simulink model "p2Sim"  (R2020a)
settings: Solver=ode3  StartTime=0.0  StopTime=simPrm.tEnd  FixedStep=simPrm.dt  RelTol=1e-3
values from neighbouring files (symbols this model uses):
  denG = [1 4 25]    [p2Setup.m]
  denH = [Tau, 1]    [p2Setup.m]
  numG = 25    [p2Setup.m]
  numH = 1    [p2Setup.m]
  Umax = 2.5    [p2Setup.m]
  Umin = -2.5    [p2Setup.m]
undefined symbols (not defined in the file or in its folder): cl, Control, dend, Discrete, Input, numd, Time
libraries: simulink x1, ctrlSharedLib x1
settings Model: Creator=vmali  LastModifiedBy=vmali
settings DataIOCC: SignalLoggingName=sdata

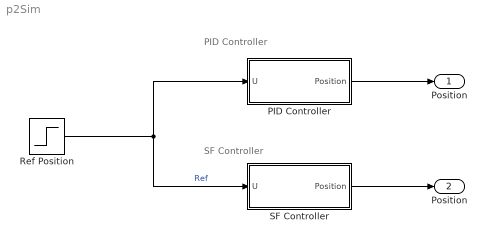
== system p2Sim ==
  note: SF Controller
  note: PID Controller
  PID Controller : Subsystem
  Ref Position : Step  Time=Input.Ts  After=Input.U  SampleTime=0
  SF Controller : Subsystem
  Position : Outport
  "Position " : Outport  Port=2
  wires:
  PID Controller/1(Position) -> Position/1
  SF Controller/1(Position) -> "Position "/1
  Ref Position/1 -> SF Controller/1(U), PID Controller/1(U)  "Ref"

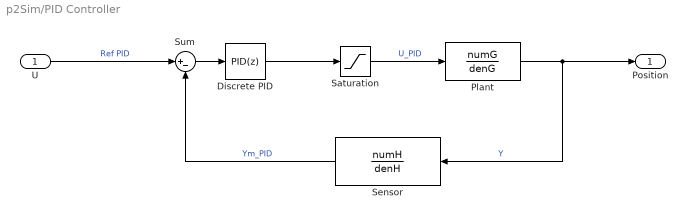
== system p2Sim/PID Controller ==
  U : Inport
  Discrete PID : simulink/Continuous/PID Controller  Controller=PID  Form=Parallel  TimeDomain=Discrete-time  UseExternalTs=off  SampleTime=Control.Z  IntegratorMethod=Forward Euler  FilterMethod=Forward Euler  ControllerParametersSource=internal  P=Control.Kp  I=Control.Ki  D=Control.Kd  UseFilter=on  N=100  TunerSelectOption=Transfer Function Based (PID Tuner App)  InitialConditionSource=internal  InitialConditionForIntegrator=0  InitialConditionForFilter=0  DifferentiatorICPrevScaledInput=0  ExternalReset=none  TrackingMode=off  Kt=1  LimitOutput=off  UpperSaturationLimit=inf  LowerSaturationLimit=-inf  LinearizeAsGain=on  AntiWindupMode=none  Kb=1  POutMin=[]  POutMax=[]  IOutMin=[]  IOutMax=[]  DOutMin=[]  DOutMax=[]  NOutMin=[]  NOutMax=[]  SumOutMin=[]  SumOutMax=[]  SaturationOutMin=[]  SaturationOutMax=[]  PParamMin=[]  PParamMax=[]  IParamMin=[]  IParamMax=[]  DParamMin=[]  DParamMax=[]  NParamMin=[]  NParamMax=[]  KbParamMin=[]  KbParamMax=[]  KtParamMin=[]  KtParamMax=[]  KbOutMin=[]  KbOutMax=[]  KtOutMin=[]  KtOutMax=[]  IntegratorOutMin=[]  IntegratorOutMax=[]  FilterOutMin=[]  FilterOutMax=[]  SumI1OutMin=[]  SumI1OutMax=[]  SumI2OutMin=[]  SumI2OutMax=[]  SumI3OutMin=[]  SumI3OutMax=[]  SumI4OutMin=[]  SumI4OutMax=[]  SumDOutMin=[]  SumDOutMax=[]  DifferentiatorOutMin=[]  DifferentiatorOutMax=[]  FilterDiffOutCoefMin=[]  FilterDiffOutCoefMax=[]  ReciprocalOutMin=[]  ReciprocalOutMax=[]  SumDenOutMin=[]  SumDenOutMax=[]  SumNumOutMin=[]  SumNumOutMax=[]  DivideOutMin=[]  DivideOutMax=[]  UdiffTsProdOutMin=[]  UdiffTsProdOutMax=[]  NTsProdOutMin=[]  NTsProdOutMax=[]  UintegralTsProdOutMin=[]  UintegralTsProdOutMax=[]  UngainTsProdOutMin=[]  UngainTsProdOutMax=[]  IntegratorContinuousStateAttributes=''  IntegratorStateMustResolveToSignalObject=off  IntegratorRTWStateStorageClass=Auto  FilterContinuousStateAttributes=''  FilterStateMustResolveToSignalObject=off  FilterRTWStateStorageClass=Auto  ParallelPVariant=InternalParameters  IdealPVariant=Disabled  IVariant=InternalParameters  DVariant=InternalParameters  IntegratorVariant=Discrete  SatVariant=Disabled  AWVariant=Passthrough  PCopyVariant=Disabled  TRVariant=Disabled  FdbkBlocksVariant=Forward  IdealPFdbkVariant=Disabled  SatFdbkVariant=Disabled  DerivativeFilterVariant=ForwardEulerFilter  NVariant=InternalParameters  NCopyVariant=Disabled  FilterICVariant=InternalICsFilter  IntegratorICVariant=InternalICs  ExternalResetVariant=Disabled  TRSumVariant=Passthrough  SumFdbkVariant=Disabled  SumVariant=Sum_PID  TsampFilterVariant=InternalTs  TsampNgainVariant=Passthrough  TsampIntegralVariant=Passthrough
  Plant : TransferFcn  Numerator=numG  Denominator=denG
  Saturation : Saturate  UpperLimit=Umax  LowerLimit=Umin
  Sensor : TransferFcn  Numerator=numH  Denominator=denH
  Sum : Sum  Inputs=|+-
  Position : Outport
  wires:
  Plant/1 -> Sensor/1, Position/1  "Y"
  Sensor/1 -> Sum/2  "Ym_PID"
  Sum/1 -> Discrete PID/1
  Saturation/1 -> Plant/1  "U_PID"
  Discrete PID/1 -> Saturation/1
  U/1 -> Sum/1  "Ref PID"

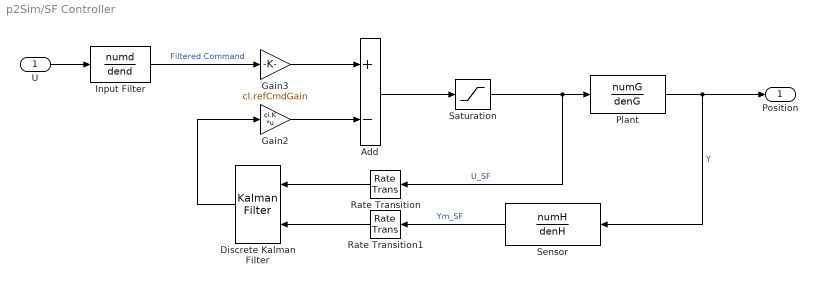
== system p2Sim/SF Controller ==
  U : Inport
  Add : Sum  Inputs=+-
  Discrete Kalman Filter : ctrlSharedLib/Kalman Filter  TimeDomain=Discrete-Time  UseCurrentEstimator=on  ModelSource=LTI State-Space Variable  ModelSourceVariable=P.ssd  A=0.95  B=1  C=1  D=0  NumberOfStates=1  NumberOfInputs=1  NumberOfOutputs=1  InitialEstimateSource=Dialog  X0=0  P0=10  UseK=off  UseGH=off  NumberOfProcessNoiseInputs=1  G=1  TimeInvariantG=on  H=0  TimeInvariantH=on  Q=0.05  TimeInvariantQ=on  R=1  TimeInvariantR=on  N=0  TimeInvariantN=on  AddInputPort=on  AddEnablePort=off  OutputEstimatedY=off  OutputP=off  Ts=-1
  Gain2 : Gain  Gain=cl.K  Multiplication=Matrix(K*u)
      settings: AttributesFormatString=%<Gain>
  Gain3 : Gain  Gain=cl.refCmdGain
      settings: AttributesFormatString=%<Gain>
  Input Filter : DiscreteTransferFcn  Numerator=numd  Denominator=dend  SampleTime=Control.Z
  Plant : TransferFcn  Numerator=numG  Denominator=denG
  Rate Transition : RateTransition  OutPortSampleTime=Control.Z
  Rate Transition1 : RateTransition  OutPortSampleTime=Control.Z
  Saturation : Saturate  UpperLimit=Umax  LowerLimit=Umin
  Sensor : TransferFcn  Numerator=numH  Denominator=denH
  Position : Outport
  wires:
  Gain2/1 -> Add/2
  Gain3/1 -> Add/1
  Rate Transition/1 -> Discrete Kalman Filter/1
  Plant/1 -> Sensor/1, Position/1  "Y"
  Sensor/1 -> Rate Transition1/1  "Ym_SF"
  Rate Transition1/1 -> Discrete Kalman Filter/2
  Saturation/1 -> Rate Transition/1, Plant/1  "U_SF"
  U/1 -> Input Filter/1
  Add/1 -> Saturation/1
  Discrete Kalman Filter/1 -> Gain2/1
  Input Filter/1 -> Gain3/1  "Filtered Command"
